simulink model "Closed_loop_control"  (R2023b)
settings: Solver=VariableStepAuto  StartTime=0.0  StopTime=inf  RelTol=1e-3
libraries: instrumentseriallib x3, sldrtlib x1
settings Model: Creator=Badda_Bing  LastModifiedBy=Badda_Bing

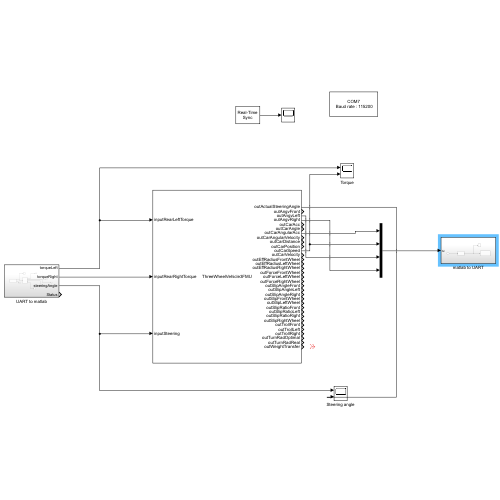
[thumbnail: Simulink's stored preview of the top-level diagram]
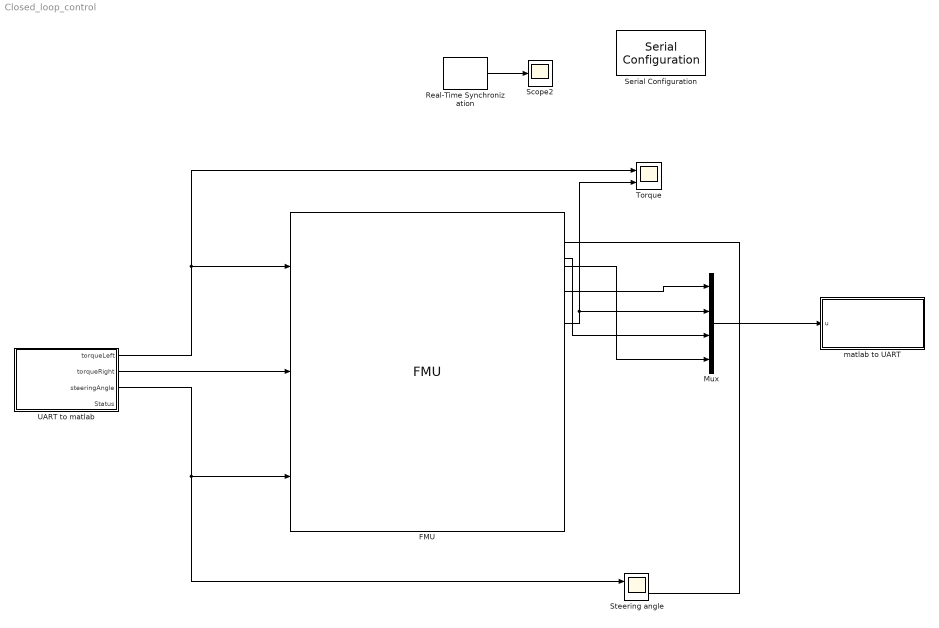
== system Closed_loop_control ==
  FMU : FMU  FMUName=ThreeWheelVehicle3FMUpid.fmu  FMUMode=ModelExchange  FMUInitializeEnumObject=off  airResistanceLongitudinal=struct('r',[0.0,1.0],'rho',1.18)  backLength=0.5  body2=struct('I',1e-08,'m',0.1)  c_rollF=0.05  c_rollL=0.05  c_rollR=0.05  dragCoef=0.5  front=struct('r',[0.0],'width',0.2)  front2=struct('r',[1e-10,0.0])  frontLength=1.5  frontTrail=struct('r',[0.0,-0.1])  frontWheel=struct('diameter',0.1,'r',[0.0,1.0],'v0_roll',0.1)  g=9.82  gearRatio=0.125  inertiaBody=350.0  inertiaWheelF=0.3  inertiaWheelL=0.3  inertiaWheelR=0.3  mass=350.0  massCenterZ=0.3  muAF=1.0  muAL=1.0  muAR=1.0  muSF=0.7  muSL=0.7  muSR=0.7  neg=struct('k',-1.0)  neg2=struct('k',-1.0)  planarWorld=struct('constantGravity',[0.0,0.0],'defaultFrameDiameterFraction',40.0,'defaultN_to_m',1000.0,'defaultNm_to_m',1000.0,'defaultSpecularCoefficient',0.7,'defaultWidthFraction',20.0,'defaultZPosition',0.0,'gravityArrowTail',[0.0,0.0],'nominalLength',1.0)  positionPhi=struct('f_crit',50.0)  rear=struct('r',[0.0],'width',0.2)  rearLeft=struct('r',[0,0.0])  rearLeftWheel=struct('diameter',0.1,'r',[0.0,1.0],'v0_roll',0.1)  rearRight=struct('r',[0,0.0])  rearRightWheel=struct('diameter',0.1,'r',[0.0,1.0],'v0_roll',0.1)  sAdF=0.07000000000000001  sAdL=0.07000000000000001  sAdR=0.07000000000000001  sSlF=0.2  sSlL=0.2  sSlR=0.2  speedStart=11.11111111111111  turnRadiusMAX=1000.0  vAdF=0.1  vAdL=0.1  vAdR=0.1  vSlF=0.3  vSlL=0.3  vSlR=0.3  vehicleFrontArea=1.5  vehicleWidth=1.0  wheelRadiusF=0.28  wheelRadiusL=0.28  wheelRadiusR=0.28  body_sphere_shapeType=sphere  body2_sphere_shapeType=sphere  front_cylinder_shapeType=cylinder  front2_cylinder_shapeType=cylinder  frontTrail_cylinder_shapeType=cylinder  frontWheel_cylinder_shapeType=cylinder  frontWheel_rim1_shapeType=cylinder  frontWheel_rim2_shapeType=cylinder  planarWorld_label1=x  planarWorld_label2=y  rear_cylinder_shapeType=cylinder  rearLeft_cylinder_shapeType=cylinder  rearLeftWheel_cylinder_shapeType=cylinder  rearLeftWheel_rim1_shapeType=cylinder  rearLeftWheel_rim2_shapeType=cylinder  rearRight_cylinder_shapeType=cylinder  rearRightWheel_cylinder_shapeType=cylinder  rearRightWheel_rim1_shapeType=cylinder  rearRightWheel_rim2_shapeType=cylinder  revolute_cylinder_shapeType=cylinder  mask(ThreeWheelVehicle3FMU [Model Exchange, v2.0]){}
      settings: MultithreadedSim=off
      mask Display:
      | disp('ThreeWheelVehicle3FMU');
      | port_label('output',1,'outActualSteeringAngle');
      | port_label('output',2,'outAngvFront');
      | port_label('output',3,'outAngvLeft');
      | port_label('output',4,'outAngvRight');
      | port_label('output',5,'outCarAcc');
      | port_label('output',6,'outCarAngle');
      | port_label('output',7,'outCarAngularAcc');
      | port_label('output',8,'outCarAngularVelocity');
      | port_label('output',9,'outCarDistance');
      | port_label('output',10,'outCarPosition');
      | port_label('output',11,'outCarSpeed');
      | port_label('output',12,'outCarVelocity');
      | port_label('output',13,'outEffRadiusFrontWheel');
      | port_label('output',14,'outEffRadiusLeftWheel');
      | port_label('output',15,'outEffRadiusRightWheel');
      | port_label('output',16,'outForceFrontWheel');
      | port_label('output',17,'outForceLeftWheel');
      | port_label('output',18,'outForceRightWheel');
      | port_label('output',19,'outSlipAngleFront');
      | port_label('output',20,'outSlipAngleLeft');
      | port_label('output',21,'outSlipAngleRight');
      | port_label('output',22,'outSlipFrontWheel');
      | port_label('output',23,'outSlipLeftWheel');
      | port_label('output',24,'outSlipRatioFront');
      | port_label('output',25,'outSlipRatioLeft');
      | port_label('output',26,'outSlipRatioRight');
      | port_label('output',27,'outSlipRightWheel');
      | port_label('output',28,'outTrollFront');
      | port_label('output',29,'outTrollLeft');
      | port_label('output',30,'outTrollRight');
      | port_label('output',31,'outTurnRadOptimal');
      | port_label('output',32,'outTurnRadReal');
      | port_label('output',33,'outWeightTransfer');
      | port_label('input',1,'inputRearLeftTorque');
      | port_label('input',2,'inputRearRightTorque');
      | port_label('input',3,'inputSteering');
  Mux : Mux
  Real-Time Synchronization : sldrtlib/Real-Time Synchronization  SampleTime=0.01  MaxMissedTicks=inf  ShowMissedTicks=on  YieldWhenWaiting=off
  Scope2 : Scope
  Serial Configuration : instrumentseriallib/Serial Configuration  Priority=-200000  PortSel=COM7  Port=COM7  ComPort=COM7  BaudRate=115200  DataBits=8  Parity=none  StopBits=1  ByteOrder=little-endian  FlowControl=none  Timeout=10  SimulateUsing=Interpreted execution  BlockInModel=on  aMode=1
      settings: LibrarySourceBlock=embeddedtargetslib/Host Communication/Serial Configuration
  Steering angle : Scope  NumInputPorts=2
  Torque : Scope  NumInputPorts=2
  UART to matlab : Subsystem
  matlab to UART : Subsystem
  wires:
  Real-Time Synchronization/1 -> Scope2/1
  ? -> ?
  UART to matlab/1(torqueLeft) -> FMU/1, Torque/1
  UART to matlab/2(torqueRight) -> FMU/2
  UART to matlab/3(steeringAngle) -> FMU/3, Steering angle/1
  FMU/1 -> Steering angle/2
  FMU/11 -> Mux/2, Torque/2
  FMU/4 -> Mux/4
  Mux/1 -> matlab to UART/1(u)
  FMU/7 -> Mux/1
  FMU/3 -> Mux/3

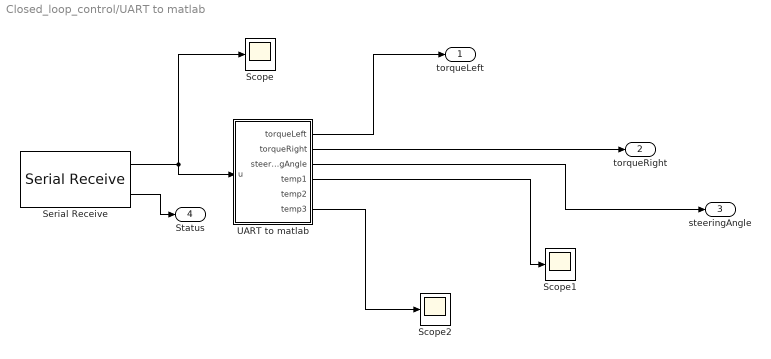
== system Closed_loop_control/UART to matlab ==
  Scope : Scope
  Scope1 : Scope
  Scope2 : Scope
  Serial Receive : instrumentseriallib/Serial Receive  Priority=1  PortSel=COM7  Port=COM7  ComPort=COM7  DataType=uint8  SaveDataType=uint8  ToggleHeader=off  Header=[]  ToggleTerminator=off  Terminator=<none>  CustomTerminator=[]  InputFormat=Column major  ToggleDataSize=on  DataSize=[1 12]  EnableBlockingMode=off  ActionDataUnavailable=Output last received value  ActionWhenDataUnavailable=Output last received value  CustomValue=0  SampleTime=0.01  SimulateUsing=Interpreted execution  BlockInModel=on  aMode=1
      settings: LibrarySourceBlock=embeddedtargetslib/Host Communication/Serial Receive
  UART to matlab : MATLAB Function  TreatAsAtomicUnit=on
  torqueLeft : Outport  OutDataTypeStr=double
  torqueRight : Outport  Port=2  OutDataTypeStr=double
  steeringAngle : Outport  Port=3  OutDataTypeStr=double
  Status : Outport  Port=4
  wires:
  Serial Receive/1 -> Scope/1, UART to matlab/1(u)
  UART to matlab/3(steeringAngle) -> steeringAngle/1
  UART to matlab/2(torqueRight) -> torqueRight/1
  UART to matlab/1(torqueLeft) -> torqueLeft/1
  Serial Receive/2 -> Status/1
  UART to matlab/4(temp1) -> Scope1/1
  UART to matlab/6(temp3) -> Scope2/1

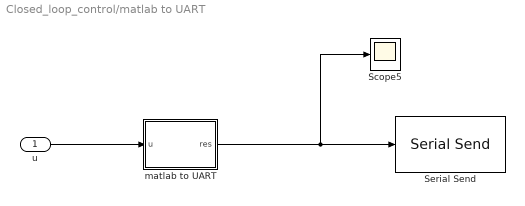
== system Closed_loop_control/matlab to UART ==
  u : Inport
  Scope5 : Scope
  Serial Send : instrumentseriallib/Serial Send  Priority=1  PortSel=COM7  Port=COM7  ComPort=COM7  Header=[]  Terminator=<none>  CustomTerminator=[]  EnableBlockingMode=off  SimulateUsing=Interpreted execution  BlockInModel=on  aMode=1
      settings: LibrarySourceBlock=embeddedtargetslib/Host Communication/Serial Send
  matlab to UART : MATLAB Function  TreatAsAtomicUnit=on
  wires:
  matlab to UART/1(res) -> Scope5/1, Serial Send/1
  u/1 -> matlab to UART/1(u)

== matlab function Closed_loop_control/UART to matlab/UART to matlab ==
  data: u input uint8 size=[1,12]; torqueLeft output double; torqueRight output double; steeringAngle output double; temp1 output; temp2 output; temp3 output
function [torqueLeft, torqueRight, steeringAngle, temp1, temp2, temp3] = fcn(u)
    temp1 = flip(u(1:4));
    torqueLeft = cast(typecast(temp1, "single"), "double");
    temp2 = flip(u(5:8));
    torqueRight = cast(typecast(temp2, "single"), "double");
    temp3 = flip(u(9:12));
    steeringAngle = cast(typecast(temp3, "single"), "double");
end

== matlab function Closed_loop_control/matlab to UART/matlab to UART ==
  data: u input double size=[1, 5]; res output uint8 size=[1, 20]
function res = fcn(u)
temp1 = cast(u(1), "single");
angularAcc = flip(typecast(temp1, "uint8_t"));
temp2 = cast(u(2), "single");
vX = flip(typecast(temp2, "uint8_t"));
temp3 = cast(u(3), "single");
angularVelocityLeftWheel = flip(typecast(temp3, "uint8_t"));
temp4 = cast(u(4), "single");
angularVelocityRightWheel = flip(typecast(temp4, "uint8_t"));

res = [angularAcc, vX, angularVelocityLeftWheel, angularVelocityRightWheel];
